simulink model "heli_obs"  (R2021a)
settings: Solver=VariableStepAuto  StartTime=0.0  StopTime=10  FixedStep=0.001  RelTol=1e-3
values from neighbouring files (symbols this model uses):
  A = [-0.4 0 -0.01 ... (first row only)    [heli.m]
  B = [6.3 0 9.8]'    [heli.m]
  C = [0 0 1]    [heli.m]
  E = [eval(ESO.E1) eval(ESO.E2) eval(ESO.E3)]'    [heli.m]
  K = [eval(KSO.K1) eval(KSO.K2) eval(KSO.K3)]    [heli.m]
settings Model: Creator=McQueen_Zero  LastModifiedBy=McQueen_Zero
settings OptimizationCC: DefaultParameterBehavior=Inlined  BufferReuse=off
settings DebuggingCC: InitInArrayFormatMsg=none

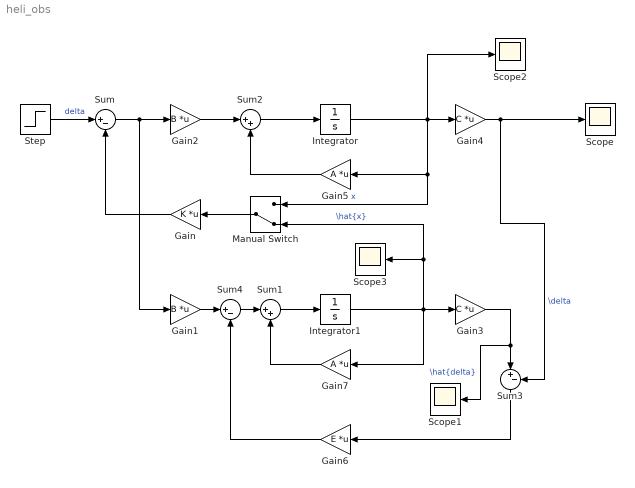
== system heli_obs ==
  Gain : Gain  Gain=K  Multiplication=Matrix(K*u)
  Gain1 : Gain  Gain=B  Multiplication=Matrix(K*u)
  Gain2 : Gain  Gain=B  Multiplication=Matrix(K*u)
  Gain3 : Gain  Gain=C  Multiplication=Matrix(K*u)
  Gain4 : Gain  Gain=C  Multiplication=Matrix(K*u)
  Gain5 : Gain  Gain=A  Multiplication=Matrix(K*u)
  Gain6 : Gain  Gain=E  Multiplication=Matrix(K*u)
  Gain7 : Gain  Gain=A  Multiplication=Matrix(K*u)
  Integrator : Integrator
  Integrator1 : Integrator
  Manual Switch : ManualSwitch  CurrentSetting=0
  Scope{,1..3} (4 alike) : Scope
  Step : Step  Time=0  SampleTime=0
  Sum : Sum  Inputs=|+-
  Sum1 : Sum  Inputs=|++
  Sum2 : Sum  Inputs=|++
  Sum3 : Sum  Inputs=|+-
  Sum4 : Sum  Inputs=|+-
  wires:
  Integrator/1 -> Gain4/1, Scope2/1, Manual Switch/1, Gain5/1  "x"
  Step/1 -> Sum/1  "delta"
  Manual Switch/1 -> Gain/1
  Gain/1 -> Sum/2
  Gain2/1 -> Sum2/1
  Sum2/1 -> Integrator/1
  Gain4/1 -> Sum3/2, Scope/1  "\\delta"
  Gain5/1 -> Sum2/2
  Gain1/1 -> Sum4/1
  Integrator1/1 -> Scope3/1, Manual Switch/2, Gain3/1, Gain7/1  "\\hat{x}"
  Sum/1 -> Gain1/1, Gain2/1
  Gain7/1 -> Sum1/2
  Sum1/1 -> Integrator1/1
  Gain3/1 -> Sum3/1, Scope1/1  "\\hat{delta}"
  Sum3/1 -> Gain6/1
  Sum4/1 -> Sum1/1
  Gain6/1 -> Sum4/2
